simulink model "block_diagram_for_single_phase_vsi"  (R2014a)
settings: Solver=ode23t  StartTime=0.0  StopTime=1  MaxStep=1e-6  RelTol=1e-3
values from neighbouring files (symbols this model uses):
  p11 = rem(m,360)    [code_for_single_phase_csi.m]    (also in code_for_single_phase_vsi.m; code_for_three_phase_csi.m; code_for_three_phase_vsi.m; code_for_vsi.m)
  p22 = rem(n,360)    [code_for_single_phase_csi.m]    (also in code_for_single_phase_vsi.m; code_for_three_phase_csi.m; code_for_three_phase_vsi.m; code_for_vsi.m)
  p33 = rem(o,360)    [code_for_single_phase_csi.m]    (also in code_for_single_phase_vsi.m; code_for_three_phase_csi.m; code_for_three_phase_vsi.m; code_for_vsi.m)
  p44 = rem(p,360)    [code_for_single_phase_csi.m]    (also in code_for_single_phase_vsi.m; code_for_three_phase_csi.m; code_for_three_phase_vsi.m; code_for_vsi.m)
  p55 = rem(q,360)    [code_for_single_phase_csi.m]    (also in code_for_single_phase_vsi.m; code_for_three_phase_csi.m; code_for_three_phase_vsi.m; code_for_vsi.m)
  p66 = rem(r,360)    [code_for_single_phase_csi.m]    (also in code_for_single_phase_vsi.m; code_for_three_phase_csi.m; code_for_three_phase_vsi.m; code_for_vsi.m)
  p77 = rem(s,360)    [code_for_single_phase_csi.m]    (also in code_for_single_phase_vsi.m; code_for_three_phase_csi.m; code_for_three_phase_vsi.m; code_for_vsi.m)
libraries: powerlib x11, powerlib_meascontrol x2
settings Model: Creator=singa  LastModifiedBy=singa

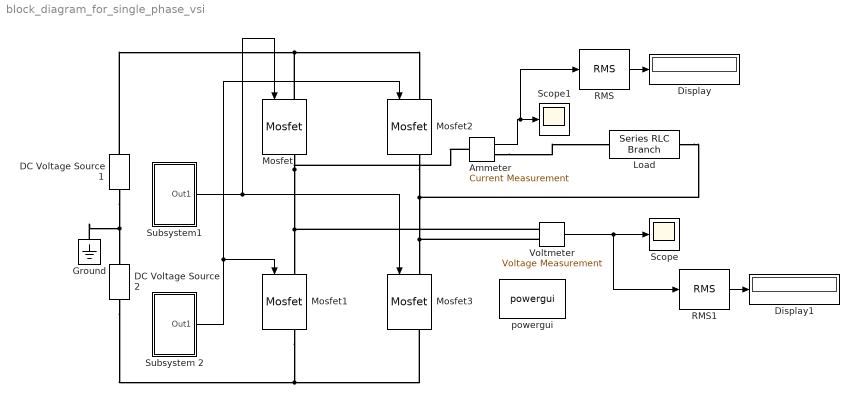
== system block_diagram_for_single_phase_vsi ==
  Ammeter : powerlib/Measurements/Current Measurement  PhasorSimulation=off  OutputType=Complex  PSBequivalent=0
  DC Voltage Source 1 : powerlib/Electrical Sources/DC Voltage Source  Amplitude=100  Measurements=None
  DC Voltage Source 2 : powerlib/Electrical Sources/DC Voltage Source  Amplitude=100  Measurements=None
  Display : Display
  Display1 : Display
  Ground : powerlib/Elements/Ground  LConnTagsString=a
  Load : powerlib/Elements/Series RLC Branch  LConnTagsString=__new0  RConnTagsString=__new0  BranchType=RL  Resistance=10  Inductance=0.05  SetiL0=off  InitialCurrent=0  Capacitance=1e-6  Setx0=off  InitialVoltage=0  Measurements=None
  Mosfet{,1..3} (4 alike) : powerlib/Power Electronics/Mosfet  Ron=0.1  Lon=0  Rd=0.01  Vfd=0  IC=0  Rs=1e5  Cs=inf  Measurements=on
  RMS : powerlib_meascontrol/Measurements/RMS  TrueRMS=on  Freq=50  RMSInit=120  Ts=0
  RMS1 : powerlib_meascontrol/Measurements/RMS  TrueRMS=on  Freq=50  RMSInit=120  Ts=0
  Scope : Scope
      settings: YMin=-800  YMax=800  SaveName=line_voltage  SampleInput=on  SampleTime=1e-6
  Scope1 : Scope
      settings: YMin=-800  YMax=800  SaveName=current  SampleInput=on  SampleTime=1e-6
  Subsystem 2 : Subsystem
  Subsystem1 : Subsystem
  Voltmeter : powerlib/Measurements/Voltage Measurement  PhasorSimulation=off  OutputType=Complex  PSBequivalent=0
  powergui : powerlib/powergui  Priority=1  SimulationMode=Continuous  SolverType=Tustin  SampleTime=50e-6  frequency=60  SPID=off  DisableSnubberDevices=off  DisableRonSwitches=off  DisableVfSwitches=off  SwTol=0  Interpol=off  DisplayEquations=off  Ts=0  methode=off  frequencyindice=0  Pbase=100e6  ErrMax=1e-4  Iterations=50  UnitsV=kV  UnitsW=MW  FunctionMessages=off  echomessages=off  HookPort=off  EnableUseOfTLC=off  x0status=blocks  RestoreLinks=warning  ResistiveCurrentMeasurement=off  Frange=[0:2:500]  Ylog=off  Xlog=on  ShowGrid=off  save=off  variable=ZData  structure=current  ZoomFFT=off  StartTime=0.8  cycles=2  DisplayStyle=4  fundamental=50  FreqAxis=on  MaxFrequency=2000  frequencyindicesteady=1  RmsSteady=1  display=off
  wires:
  Ammeter/1 -> RMS/1, Scope1/1
  Subsystem 2/1(Out1) -> Mosfet2/1, Mosfet1/1
  Subsystem1/1(Out1) -> Mosfet3/1, Mosfet/1
  RMS/1 -> Display/1
  Voltmeter/1 -> RMS1/1, Scope/1
  RMS1/1 -> Display1/1
  connections:
  DC Voltage Source 1/LConn1 -- Ground/LConn1 -- DC Voltage Source 2/RConn1
  Mosfet/RConn1 -- Voltmeter/LConn1 -- Mosfet1/LConn1 -- Ammeter/LConn1
  Mosfet2/RConn1 -- Load/RConn1 -- Voltmeter/LConn2 -- Mosfet3/LConn1
  Mosfet/LConn1 -- Mosfet2/LConn1 -- DC Voltage Source 1/RConn1
  Mosfet1/RConn1 -- Mosfet3/RConn1 -- DC Voltage Source 2/LConn1
  Ammeter/RConn1 -- Load/LConn1

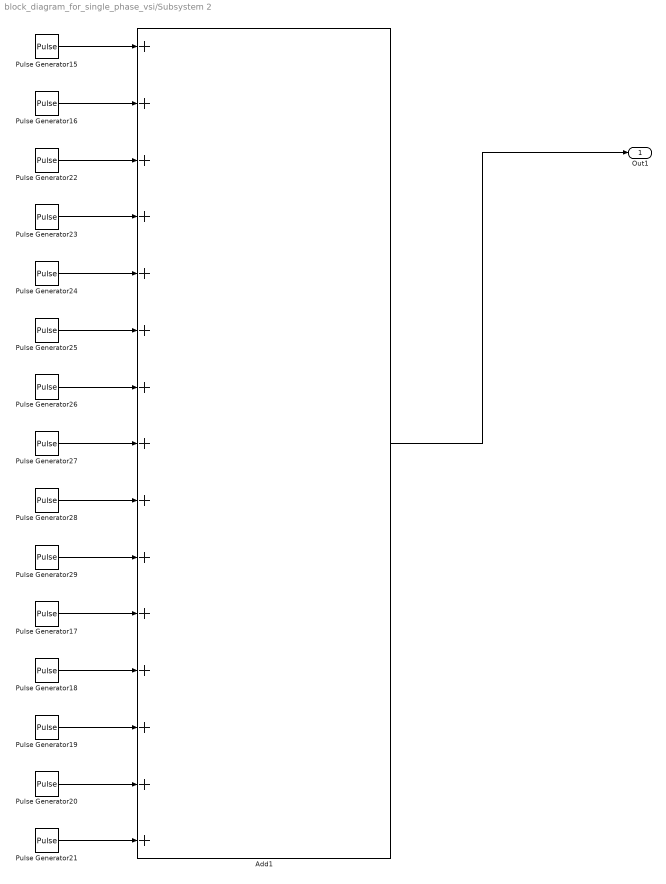
== system block_diagram_for_single_phase_vsi/Subsystem 2 ==
  Add1 : Sum  Inputs=+++++++++++++++
  Pulse Generator15 : DiscretePulseGenerator  PulseType=Time based  Period=0.02  PulseWidth=(p22-p11)/360*100  PhaseDelay=p11/360*0.02+0.01
  Pulse Generator16 : DiscretePulseGenerator  PulseType=Time based  Period=0.02  PulseWidth=(p44-p33)/360*100  PhaseDelay=p33/360*0.02+0.01
  Pulse Generator17 : DiscretePulseGenerator  PulseType=Time based  Period=0.02  PulseWidth=(p77-p66)/360*100  PhaseDelay=(180+p66)/360*0.02+0.01
  Pulse Generator18 : DiscretePulseGenerator  PulseType=Time based  Period=0.02  PulseWidth=(p77-p66)/360*100  PhaseDelay=(360-p77)/360*0.02+0.01
  Pulse Generator19 : DiscretePulseGenerator  PulseType=Time based  Period=0.02  PulseWidth=(p55-p44)/360*100  PhaseDelay=(360-p55)/360*0.02+0.01
  Pulse Generator20 : DiscretePulseGenerator  PulseType=Time based  Period=0.02  PulseWidth=(p33-p22)/360*100  PhaseDelay=(360-p33)/360*0.02+0.01
  Pulse Generator21 : DiscretePulseGenerator  PulseType=Time based  Period=0.02  PulseWidth=(p11)/360*100  PhaseDelay=(360-p11)/360*0.02+0.01
  Pulse Generator22 : DiscretePulseGenerator  PulseType=Time based  Period=0.02  PulseWidth=(p66-p55)/360*100  PhaseDelay=p55/360*0.02+0.01
  Pulse Generator23 : DiscretePulseGenerator  PulseType=Time based  Period=0.02  PulseWidth=(90-p77)/180*100  PhaseDelay=p77/360*0.02+0.01
  Pulse Generator24 : DiscretePulseGenerator  PulseType=Time based  Period=0.02  PulseWidth=(p66-p55)/360*100  PhaseDelay=(180-p66)/360*0.02+0.01
  Pulse Generator25 : DiscretePulseGenerator  PulseType=Time based  Period=0.02  PulseWidth=(p44-p33)/360*100  PhaseDelay=(180-p44)/360*0.02+0.01
  Pulse Generator26 : DiscretePulseGenerator  PulseType=Time based  Period=0.02  PulseWidth=(p22-p11)/360*100  PhaseDelay=(180-p22)/360*0.02+0.01
  Pulse Generator27 : DiscretePulseGenerator  PulseType=Time based  Period=0.02  PulseWidth=(p11)/360*100  PhaseDelay=(180)/360*0.02+0.01
  Pulse Generator28 : DiscretePulseGenerator  PulseType=Time based  Period=0.02  PulseWidth=(p33-p22)/360*100  PhaseDelay=(180+p22)/360*0.02+0.01
  Pulse Generator29 : DiscretePulseGenerator  PulseType=Time based  Period=0.02  PulseWidth=(p55-p44)/360*100  PhaseDelay=(180+p44)/360*0.02+0.01
  Out1 : Outport
  wires:
  Pulse Generator15/1 -> Add1/1
  Pulse Generator16/1 -> Add1/2
  Pulse Generator22/1 -> Add1/3
  Pulse Generator23/1 -> Add1/4
  Pulse Generator24/1 -> Add1/5
  Pulse Generator25/1 -> Add1/6
  Pulse Generator26/1 -> Add1/7
  Pulse Generator27/1 -> Add1/8
  Pulse Generator19/1 -> Add1/13
  Pulse Generator29/1 -> Add1/10
  Add1/1 -> Out1/1
  Pulse Generator20/1 -> Add1/14
  Pulse Generator17/1 -> Add1/11
  Pulse Generator28/1 -> Add1/9
  Pulse Generator18/1 -> Add1/12
  Pulse Generator21/1 -> Add1/15

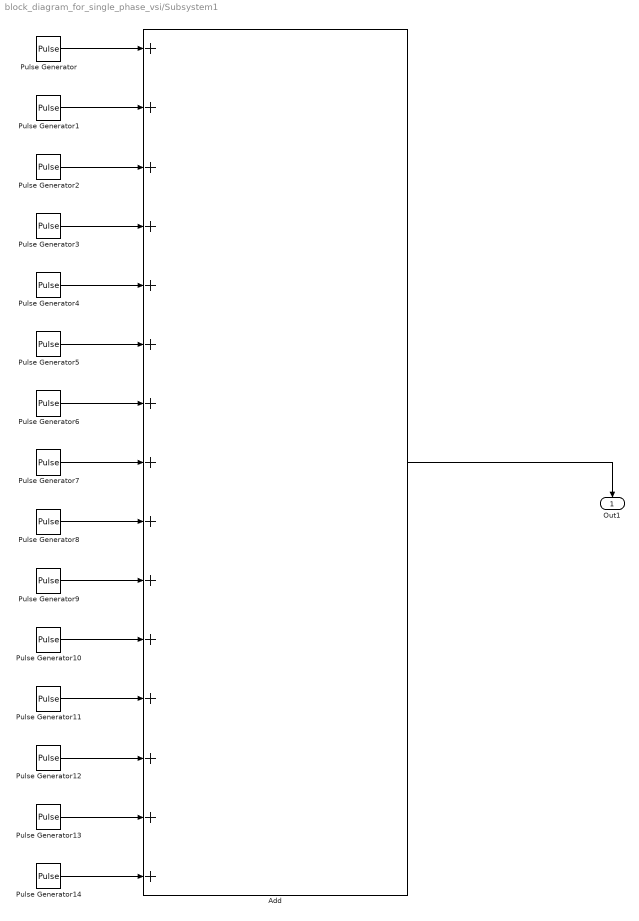
== system block_diagram_for_single_phase_vsi/Subsystem1 ==
  Add : Sum  Inputs=+++++++++++++++
  Pulse Generator : DiscretePulseGenerator  PulseType=Time based  Period=0.02  PulseWidth=(p22-p11)/360*100  PhaseDelay=p11/360*0.02
  Pulse Generator1 : DiscretePulseGenerator  PulseType=Time based  Period=0.02  PulseWidth=(p44-p33)/360*100  PhaseDelay=p33/360*0.02
  Pulse Generator10 : DiscretePulseGenerator  PulseType=Time based  Period=0.02  PulseWidth=(p77-p66)/360*100  PhaseDelay=(180+p66)/360*0.02
  Pulse Generator11 : DiscretePulseGenerator  PulseType=Time based  Period=0.02  PulseWidth=(p77-p66)/360*100  PhaseDelay=(360-p77)/360*0.02
  Pulse Generator12 : DiscretePulseGenerator  PulseType=Time based  Period=0.02  PulseWidth=(p55-p44)/360*100  PhaseDelay=(360-p55)/360*0.02
  Pulse Generator13 : DiscretePulseGenerator  PulseType=Time based  Period=0.02  PulseWidth=(p33-p22)/360*100  PhaseDelay=(360-p33)/360*0.02
  Pulse Generator14 : DiscretePulseGenerator  PulseType=Time based  Period=0.02  PulseWidth=(p11)/360*100  PhaseDelay=(360-p11)/360*0.02
  Pulse Generator2 : DiscretePulseGenerator  PulseType=Time based  Period=0.02  PulseWidth=(p66-p55)/360*100  PhaseDelay=p55/360*0.02
  Pulse Generator3 : DiscretePulseGenerator  PulseType=Time based  Period=0.02  PulseWidth=(90-p77)/180*100  PhaseDelay=p77/360*0.02
  Pulse Generator4 : DiscretePulseGenerator  PulseType=Time based  Period=0.02  PulseWidth=(p66-p55)/360*100  PhaseDelay=(180-p66)/360*0.02
  Pulse Generator5 : DiscretePulseGenerator  PulseType=Time based  Period=0.02  PulseWidth=(p44-p33)/360*100  PhaseDelay=(180-p44)/360*0.02
  Pulse Generator6 : DiscretePulseGenerator  PulseType=Time based  Period=0.02  PulseWidth=(p22-p11)/360*100  PhaseDelay=(180-p22)/360*0.02
  Pulse Generator7 : DiscretePulseGenerator  PulseType=Time based  Period=0.02  PulseWidth=(p11)/360*100  PhaseDelay=(180)/360*0.02
  Pulse Generator8 : DiscretePulseGenerator  PulseType=Time based  Period=0.02  PulseWidth=(p33-p22)/360*100  PhaseDelay=(180+p22)/360*0.02
  Pulse Generator9 : DiscretePulseGenerator  PulseType=Time based  Period=0.02  PulseWidth=(p55-p44)/360*100  PhaseDelay=(180+p44)/360*0.02
  Out1 : Outport
  wires:
  Pulse Generator2/1 -> Add/3
  Pulse Generator4/1 -> Add/5
  Pulse Generator/1 -> Add/1
  Pulse Generator1/1 -> Add/2
  Pulse Generator8/1 -> Add/9
  Pulse Generator13/1 -> Add/14
  Pulse Generator14/1 -> Add/15
  Add/1 -> Out1/1
  Pulse Generator6/1 -> Add/7
  Pulse Generator11/1 -> Add/12
  Pulse Generator5/1 -> Add/6
  Pulse Generator3/1 -> Add/4
  Pulse Generator12/1 -> Add/13
  Pulse Generator9/1 -> Add/10
  Pulse Generator7/1 -> Add/8
  Pulse Generator10/1 -> Add/11
